simulink model "sobel_hdl_2018b"  (R2018b)
settings: Solver=FixedStepDiscrete  StartTime=0.0  StopTime=2200*1125  FixedStep=1  RelTol=1e-3
undefined symbols (not defined in the file or in its folder): Rec, SDTV
libraries: visionhdlio x2, visionsources x1, visionhdlconversions x1, simulink x1, visionhdlutilities x1, visionsinks x1
settings Model: SimulationMode=accelerator  Creator=linbai  LastModifiedBy=lbai
settings DataIOCC: ReturnWorkspaceOutputs=on
settings HardwareCC: ProdBitPerPointer=32  ProdBitPerSizeT=32  ProdBitPerPtrDiffT=32  ProdLargestAtomicFloat=None  ProdIntDivRoundTo=Undefined  ProdEndianess=Unspecified  ProdWordSize=32  ProdHWDeviceType=ASIC/FPGA->ASIC/FPGA  TargetBitPerPointer=64  TargetBitPerSizeT=64  TargetBitPerPtrDiffT=64  TargetLongLongMode=on  TargetIntDivRoundTo=Zero  TargetEndianess=LittleEndian  TargetWordSize=64  TargetHWDeviceType=Custom Processor->MATLAB Host Computer  ProdEqTarget=off

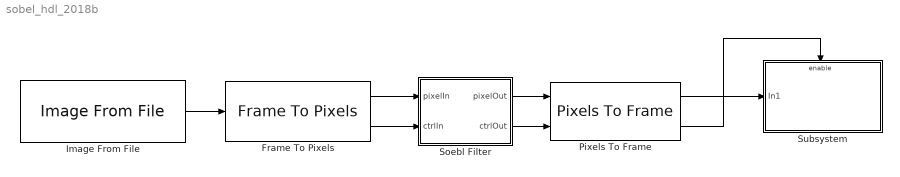
== system sobel_hdl_2018b ==
  Frame To Pixels : visionhdlio/Frame To Pixels  NumComponents=3  VideoFormat=1080p  ActivePixelsPerLine=160  ActiveVideoLines=160  TotalPixelsPerLine=400  TotalVideoLines=400  StartingActiveLine=6  FrontPorch=120  SampleTime=0
      settings: SourceProductName=Vision HDL Toolbox  SourceProductBaseCode=VT
  Image From File : visionsources/Image From File  Tag=vipblks_nd  FileName=test_1080p.bmp  Ts=2200*1125  imagePorts=One multidimensional signal  OutPortLabels=R|G|B  ImageDataType=Inherit from input image  sdImageDataType=uint(8)  Signed=on  WordLength=16  FractionLengthMode=User-defined  FractionLength=15
      settings: SourceProductName=Computer Vision Toolbox
  Pixels To Frame : visionhdlio/Pixels To Frame  NumComponents=3  VideoFormat=1080p  ActivePixelsPerLine=32  ActiveVideoLines=18  TotalPixelsPerLine=42  TotalVideoLines=28
      settings: SourceProductName=Vision HDL Toolbox  SourceProductBaseCode=VT
  Soebl Filter : Subsystem
  Subsystem : Subsystem
  wires:
  Image From File/1 -> Frame To Pixels/1
  Pixels To Frame/1 -> Subsystem/1(In1)
  Pixels To Frame/2 -> Subsystem/Enable
  Frame To Pixels/1 -> Soebl Filter/1(pixelIn)
  Frame To Pixels/2 -> Soebl Filter/2(ctrlIn)
  Soebl Filter/1(pixelOut) -> Pixels To Frame/1
  Soebl Filter/2(ctrlOut) -> Pixels To Frame/2

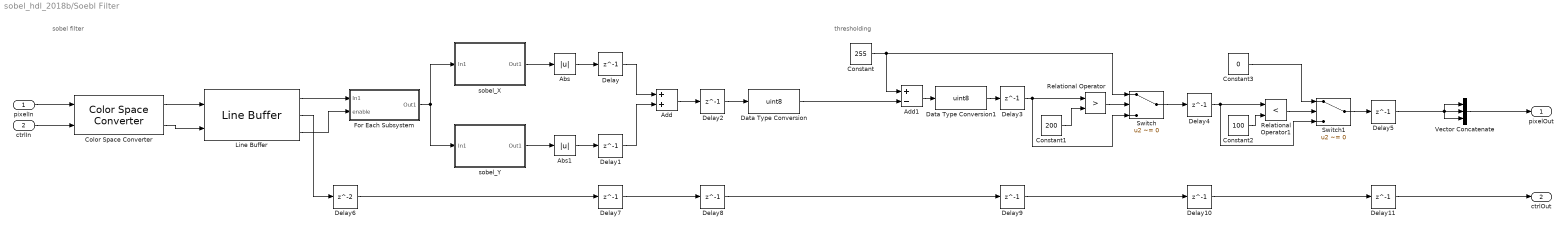
== system sobel_hdl_2018b/Soebl Filter ==
  note: thresholding
  note: sobel filter
  pixelIn : Inport
  ctrlIn : Inport  Port=2
  Abs : Abs
  Abs1 : Abs
  Add : Sum
  Add1 : Sum  Inputs=+-
  Color Space Converter : visionhdlconversions/Color Space Converter  Conversion=RGB to intensity  ConversionStandard=Rec. 601 (SDTV)  ScanningStandard=1250/50/2:1  SimulateUsing=Code generation
      settings: SourceProductName=Vision HDL Toolbox  SourceProductBaseCode=VT
  Constant : Constant  Value=255  OutDataTypeStr=uint8  SampleTime=-1
  Constant1 : Constant  Value=200  OutDataTypeStr=uint8  SampleTime=-1
  Constant2 : Constant  Value=100  OutDataTypeStr=uint8  SampleTime=-1
  Constant3 : Constant  Value=0  OutDataTypeStr=uint8  SampleTime=-1
  Data Type Conversion : DataTypeConversion  OutDataTypeStr=uint8  SaturateOnIntegerOverflow=on
  Data Type Conversion1 : DataTypeConversion  OutDataTypeStr=uint8  SaturateOnIntegerOverflow=on
  Delay{,1..5,7..11} (11 alike) : Delay  DelayLength=1
  Delay6 : Delay
  For Each Subsystem : Subsystem  TreatAsAtomicUnit=on
  Line Buffer : visionhdlutilities/Line Buffer  NeighborhoodSize=[3 3]  PaddingMethod=Symmetric  PaddingValue=0  LineBufferSize=2048  SimulateUsing=Code generation
      settings: SourceProductName=Vision HDL Toolbox  SourceProductBaseCode=VT
  Relational Operator : RelationalOperator  Operator=>  OutDataTypeStr=boolean  RndMeth=Simplest
  Relational Operator1 : RelationalOperator  Operator=<  OutDataTypeStr=boolean  RndMeth=Simplest
  Switch : Switch  Criteria=u2 ~= 0
  Switch1 : Switch  Criteria=u2 ~= 0
  Vector Concatenate : Concatenate  NumInputs=3  Mode=Multidimensional array  ConcatenateDimension=2
  sobel_X : Subsystem
  sobel_Y : Subsystem
  pixelOut : Outport  VectorParamsAs1DForOutWhenUnconnected=on
  ctrlOut : Outport  Port=2  VectorParamsAs1DForOutWhenUnconnected=on
  wires:
  Delay9/1 -> Delay10/1
  Delay10/1 -> Delay11/1
  Abs/1 -> Delay/1
  Relational Operator/1 -> Switch/2
  Delay3/1 -> Relational Operator/1, Switch/3
  Relational Operator1/1 -> Switch1/2
  Line Buffer/1 -> For Each Subsystem/1(In1)
  sobel_Y/1(Out1) -> Abs1/1
  Delay4/1 -> Relational Operator1/1, Switch1/3
  Color Space Converter/1 -> Line Buffer/1
  sobel_X/1(Out1) -> Abs/1
  Delay5/1 -> Vector Concatenate/3, Vector Concatenate/1, Vector Concatenate/2
  Add/1 -> Delay2/1
  pixelIn/1 -> Color Space Converter/1
  For Each Subsystem/1(Out1) -> sobel_X/1(In1), sobel_Y/1(In1)
  Color Space Converter/2 -> Line Buffer/2
  Constant3/1 -> Switch1/1
  Add1/1 -> Data Type Conversion1/1
  Constant/1 -> Switch/1, Add1/1
  Data Type Conversion/1 -> Add1/2
  Delay6/1 -> Delay7/1
  Line Buffer/2 -> Delay6/1
  Delay2/1 -> Data Type Conversion/1
  Delay7/1 -> Delay8/1
  Switch/1 -> Delay4/1
  Delay1/1 -> Add/2
  Vector Concatenate/1 -> pixelOut/1
  Line Buffer/3 -> For Each Subsystem/2(enable)
  Abs1/1 -> Delay1/1
  Delay8/1 -> Delay9/1
  Switch1/1 -> Delay5/1
  Delay/1 -> Add/1
  Constant2/1 -> Relational Operator1/2
  Constant1/1 -> Relational Operator/2
  Data Type Conversion1/1 -> Delay3/1
  Delay11/1 -> ctrlOut/1
  ctrlIn/1 -> Color Space Converter/2

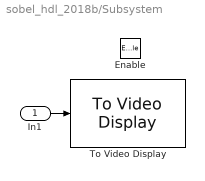
== system sobel_hdl_2018b/Subsystem ==
  In1 : Inport
  Enable : EnablePort
  To Video Display : visionsinks/To Video Display  windowSizeMode=Normal  openAtMdlStart=on  fullScreen=off  videoWindowX=0  videoWindowY=23  saveWindowSize=off  videoWindowWidth=1920  videoWindowHeight=1137  inputColorFormat=RGB  inputType=Obsolete  imagePorts=One multidimensional signal  OutputDevice=On-screen video monitor  dataOrg=Column-major  isWindowOpen=off
      settings: SourceProductName=Computer Vision Toolbox
  wires:
  In1/1 -> To Video Display/1

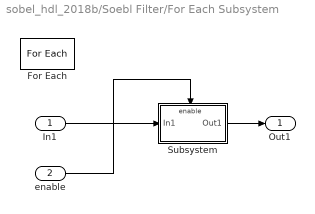
== system sobel_hdl_2018b/Soebl Filter/For Each Subsystem ==
  In1 : Inport  Partition=on  PartitionDimension=1  PartitionWidth=1  PartitionOffset=0
  enable : Inport  Port=2
  For Each : ForEach  DisableCoverage=on
  Subsystem : Subsystem
  Out1 : Outport  ConcatenationDimension=1  VectorParamsAs1DForOutWhenUnconnected=on
  wires:
  In1/1 -> Subsystem/1(In1)
  Subsystem/1(Out1) -> Out1/1
  enable/1 -> Subsystem/Enable

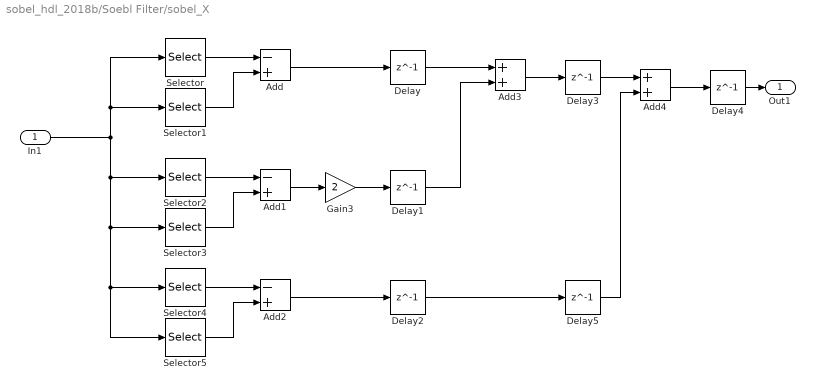
== system sobel_hdl_2018b/Soebl Filter/sobel_X ==
  In1 : Inport
  Add : Sum  Inputs=-+
  Add1 : Sum  Inputs=-+
  Add2 : Sum  Inputs=-+
  Add3 : Sum
  Add4 : Sum
  Delay{,1..5} (6 alike) : Delay  DelayLength=1
  Gain3 : Gain  Gain=2
  Selector : Selector  InputPortWidth=9  IndexOptions=Index vector (dialog)  Indices=[7]  OutputSizes=1
  Selector1 : Selector  InputPortWidth=9  IndexOptions=Index vector (dialog)  Indices=[9]  OutputSizes=1
  Selector2 : Selector  InputPortWidth=9  IndexOptions=Index vector (dialog)  Indices=[4]  OutputSizes=1
  Selector3 : Selector  InputPortWidth=9  IndexOptions=Index vector (dialog)  Indices=[6]  OutputSizes=1
  Selector4 : Selector  InputPortWidth=9  IndexOptions=Index vector (dialog)  Indices=[1]  OutputSizes=1
  Selector5 : Selector  InputPortWidth=9  IndexOptions=Index vector (dialog)  Indices=[3]  OutputSizes=1
  Out1 : Outport  VectorParamsAs1DForOutWhenUnconnected=on
  wires:
  Selector/1 -> Add/1
  Selector2/1 -> Add1/1
  Delay/1 -> Add3/1
  Gain3/1 -> Delay1/1
  In1/1 -> Selector1/1, Selector/1, Selector5/1, Selector4/1, Selector3/1, Selector2/1
  Selector1/1 -> Add/2
  Add1/1 -> Gain3/1
  Selector4/1 -> Add2/1
  Selector5/1 -> Add2/2
  Add2/1 -> Delay2/1
  Delay1/1 -> Add3/2
  Add/1 -> Delay/1
  Selector3/1 -> Add1/2
  Delay5/1 -> Add4/2
  Delay2/1 -> Delay5/1
  Delay4/1 -> Out1/1
  Add3/1 -> Delay3/1
  Delay3/1 -> Add4/1
  Add4/1 -> Delay4/1

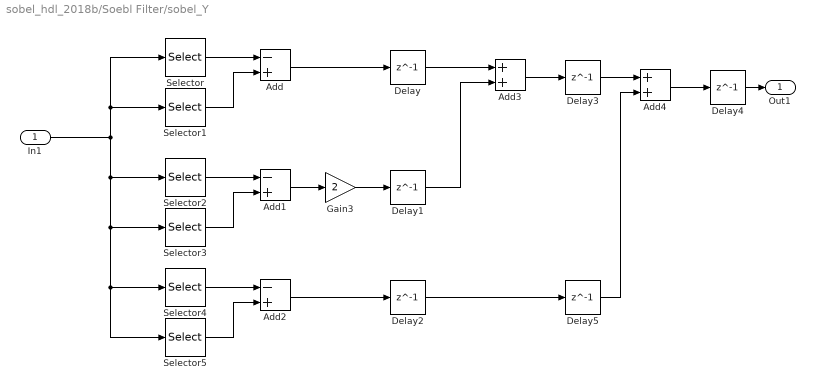
== system sobel_hdl_2018b/Soebl Filter/sobel_Y ==
  In1 : Inport
  Add : Sum  Inputs=-+
  Add1 : Sum  Inputs=-+
  Add2 : Sum  Inputs=-+
  Add3 : Sum
  Add4 : Sum
  Delay{,1..5} (6 alike) : Delay  DelayLength=1
  Gain3 : Gain  Gain=2
  Selector : Selector  InputPortWidth=9  IndexOptions=Index vector (dialog)  Indices=[1]  OutputSizes=1
  Selector1 : Selector  InputPortWidth=9  IndexOptions=Index vector (dialog)  Indices=[7]  OutputSizes=1
  Selector2 : Selector  InputPortWidth=9  IndexOptions=Index vector (dialog)  Indices=[2]  OutputSizes=1
  Selector3 : Selector  InputPortWidth=9  IndexOptions=Index vector (dialog)  Indices=[8]  OutputSizes=1
  Selector4 : Selector  InputPortWidth=9  IndexOptions=Index vector (dialog)  Indices=[3]  OutputSizes=1
  Selector5 : Selector  InputPortWidth=9  IndexOptions=Index vector (dialog)  Indices=[9]  OutputSizes=1
  Out1 : Outport  VectorParamsAs1DForOutWhenUnconnected=on
  wires:
  Add4/1 -> Delay4/1
  Delay3/1 -> Add4/1
  Add3/1 -> Delay3/1
  Delay4/1 -> Out1/1
  Delay2/1 -> Delay5/1
  Delay5/1 -> Add4/2
  Selector3/1 -> Add1/2
  Add/1 -> Delay/1
  Delay1/1 -> Add3/2
  Add2/1 -> Delay2/1
  Selector5/1 -> Add2/2
  Selector4/1 -> Add2/1
  Add1/1 -> Gain3/1
  Selector1/1 -> Add/2
  In1/1 -> Selector2/1, Selector3/1, Selector4/1, Selector5/1, Selector/1, Selector1/1
  Gain3/1 -> Delay1/1
  Delay/1 -> Add3/1
  Selector2/1 -> Add1/1
  Selector/1 -> Add/1

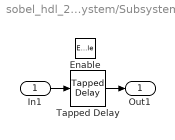
== system sobel_hdl_2018b/Soebl Filter/For Each Subsystem/Subsystem ==
  In1 : Inport
  Enable : EnablePort
  Tapped Delay : simulink/Discrete/Tapped Delay  vinit=0.0  samptime=-1  NumDelays=3  DelayOrder=Oldest  includeCurrent=off
  Out1 : Outport  VectorParamsAs1DForOutWhenUnconnected=on
  wires:
  In1/1 -> Tapped Delay/1
  Tapped Delay/1 -> Out1/1
